simulink model "Arizona_base_NI"  (R2016b)
settings: Solver=FixedStepDiscrete  StartTime=0.0  StopTime=inf  FixedStep=Ts  RelTol=1e-3  EnableMultiTasking=on
undefined symbols (not defined in the file): DiscIntNeverNeededParam, N_ref, NInit, phiInit, xInit, yInit
libraries: xpcnilib x15, simulink x9, cstblocks x3
settings Model: SimulationMode=external  ExtModeTrigDuration=5  Creator=JBolder  LastModifiedBy=Arizona
settings SolverCC: EnableConcurrentExecution=on
settings DataIOCC: LimitDataPoints=on  SaveFormat=Array
settings OptimizationCC: BlockReduction=off  OptimizeBlockIOStorage=off  BufferReuse=off  GlobalBufferReuse=off  ExpressionFolding=off  LocalBlockOutputs=off  LifeSpan=inf
settings DebuggingCC: SolverPrmCheckMsg=warning  SFUnexpectedBacktrackingDiag=warning  SFNoUnconditionalDefaultTransitionDiag=warning  SFExecutionAtInitializationDiag=none
settings HardwareCC: ProdBitPerPointer=32  ProdBitPerSizeT=32  ProdBitPerPtrDiffT=32  ProdLargestAtomicFloat=None  ProdWordSize=32  ProdLongLongMode=on  ProdHWDeviceType=Generic->32-bit x86 compatible
settings ModelReferenceCC: PropagateSignalLabelsOutOfModel=off
settings RTWCC: SystemTargetFile=slrt.tlc  TemplateMakefile=slrt_default_tmf  Description=Simulink Real-Time  CodeExecutionProfiling=on  RTWCompilerOptimization=on
settings SimulinkRealTimeCC: xPCTargetPCEnvName=ArizonaTarget
settings ConfigComp: CovMetricSettings=dw  CovHtmlReporting=on  CovSaveCumulativeToWorkspaceVar=on  CovSaveSingleToWorkspaceVar=on  CovExternalEMLEnable=off  CovSFcnEnable=off

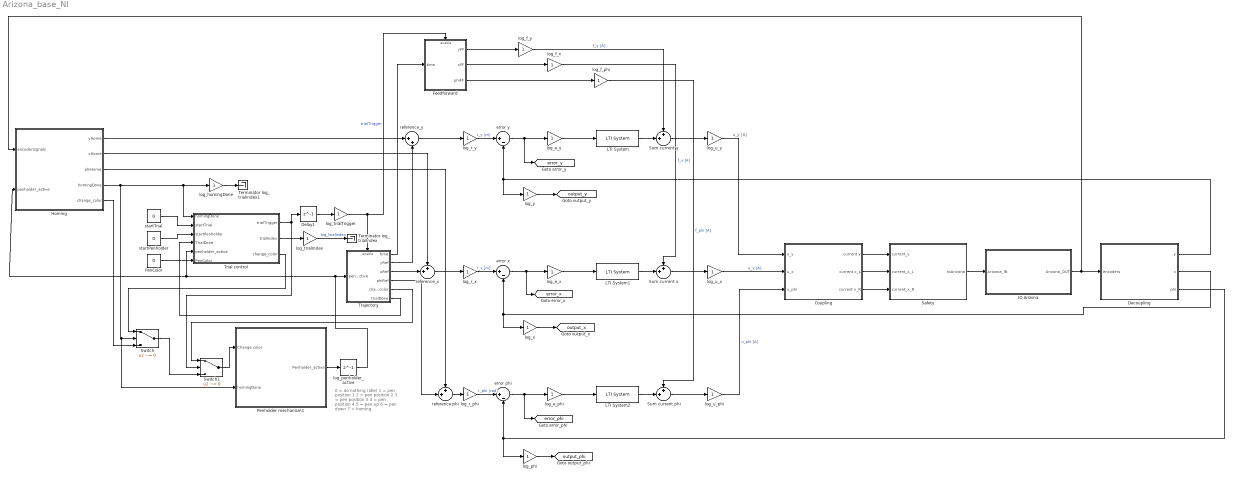
== system Arizona_base_NI ==
  note: u_y [A]
  note: 0 = do nothing (idle)
      | 1 = pen position 1
      | 2 = pen position 2
      | 3 = pen position 3
      | 4 = pen position 4
      | 5 = pen up
      | 6 = pen down
      | 7 = homing
  Coupling : Subsystem
  Decoupling : Subsystem
  Delay1 : Delay  DelayLength=1  InitialCondition=0
  Feedforward : Subsystem
  Homing : Subsystem
  IO Arizona : Subsystem
  LTI System : cstblocks/LTI System  sys=Cy  IC=[]
  LTI System1 : cstblocks/LTI System  sys=Cx  IC=[]
  LTI System2 : cstblocks/LTI System  sys=Cphi  IC=[]
  PenColor : Constant  Value=0
  Penholder mechanism1 : Subsystem
  Safety : Subsystem
  Sum current phi : Sum  Inputs=++|
  Sum current x : Sum  Inputs=++|
  Sum current y : Sum  Inputs=++|
  Switch : Switch  Criteria=u2 ~= 0
  Switch1 : Switch  Criteria=u2 ~= 0
  Terminator log_trialIndex : Terminator
  Terminator log_trialIndex1 : Terminator
  Trajectory : Subsystem  TreatAsAtomicUnit=on
  Trial control : Stateflow chart  TreatAsAtomicUnit=on
  error phi : Sum  Inputs=|+-
  error x : Sum  Inputs=|+-
  error y : Sum  Inputs=|+-
  log_e_phi : Gain
  log_e_x : Gain
  log_e_y : Gain
  log_f_phi : Gain
  log_f_x : Gain
  log_f_y : Gain
  log_homingDone : Gain
  log_penholder_active : Delay  DelayLength=1  InitialCondition=0
  log_phi : Gain
  log_r_phi : Gain
  log_r_x : Gain
  log_r_y : Gain
  log_trialIndex : Gain
  log_trialTrigger : Gain
  log_u_phi : Gain
  log_u_x : Gain
  log_u_y : Gain
  log_x : Gain
  log_y : Gain
  reference phi : Sum  Inputs=++|
  reference_x : Sum  Inputs=++|
  reference_y : Sum  Inputs=|++
  startPenholder : Constant  Value=0
  startTrial : Constant  Value=0
  tag scope: error_phi=global, error_x=global, error_y=global, output_phi=global, output_x=global, output_y=global
  wires:
  Decoupling/2(x) -> log_x/1, error x/2
  error x/1 -> log_e_x/1, [error_x]
  IO Arizona/1(Arizona_OUT) -> Decoupling/1(encoders), Homing/1(encoderSignals)
  error phi/1 -> log_e_phi/1, [error_phi]
  Homing/1(yHome) -> reference_y/1
  reference_y/1 -> log_r_y/1
  reference_x/1 -> log_r_x/1
  reference phi/1 -> log_r_phi/1
  Safety/1(toArizona) -> IO Arizona/1(Arizona_IN)
  Sum current phi/1 -> log_u_phi/1
  Trajectory/2(yRef) -> reference_y/2
  Trajectory/3(xRef) -> reference_x/2
  Trajectory/4(phiRef) -> reference phi/2
  error y/1 -> log_e_y/1, [error_y]
  Homing/3(phiHome) -> reference phi/1
  Homing/2(xHome) -> reference_x/1
  Homing/4(homingDone) -> Trial control/1(homingDone), log_homingDone/1, Penholder mechanism1/2(homingDone), Switch/2
  Trial control/1(trialTrigger) -> Switch1/2, Delay1/1
  startTrial/1 -> Trial control/2(startTrial)
  Trial control/2(trialIndex) -> log_trialIndex/1
  log_trialIndex/1 -> Terminator log_trialIndex/1  "log_trialIndex"
  log_trialTrigger/1 -> Feedforward/Enable, Trajectory/Enable  "trialTrigger"
  Feedforward/1(yFF) -> log_f_y/1
  log_e_y/1 -> LTI System/1
  Sum current y/1 -> log_u_y/1
  log_homingDone/1 -> Terminator log_trialIndex1/1
  log_r_y/1 -> error y/1  "r_y [m]"
  log_f_y/1 -> Sum current y/1  "f_y [A]"
  Feedforward/2(xFF) -> log_f_x/1
  log_f_x/1 -> Sum current x/1  "f_x [A]"
  log_r_x/1 -> error x/1  "r_x [m]"
  log_r_phi/1 -> error phi/1  "r_phi [rad]"
  log_f_phi/1 -> Sum current phi/1  "f_phi [A]"
  Feedforward/3(phiFF) -> log_f_phi/1
  log_u_y/1 -> Coupling/1(u_y)
  Sum current x/1 -> log_u_x/1
  Coupling/2(current x_L) -> Safety/2(current_x_L)
  Coupling/3(current x_R) -> Safety/3(current_x_R)
  Coupling/1(current y) -> Safety/1(current_y)
  Decoupling/1(y) -> log_y/1, error y/2
  Decoupling/3(phi) -> log_phi/1, error phi/2
  log_u_x/1 -> Coupling/2(u_x)  "u_x [A]"
  log_u_phi/1 -> Coupling/3(u_phi)  "u_phi [A]"
  log_penholder_active/1 -> Trajectory/1(penholder_active), Homing/2(penholder_active), Trial control/5(penholder_active)
  Trajectory/1(time) -> Feedforward/1(time)
  startPenholder/1 -> Trial control/3(startPenholder)
  Homing/5(change_color) -> Switch/3
  Switch1/1 -> Penholder mechanism1/1(Change color)
  Switch/1 -> Switch1/3
  Trajectory/6(trialDone) -> Trial control/4(TrialDone)
  Penholder mechanism1/1(Penholder_active) -> log_penholder_active/1
  Delay1/1 -> log_trialTrigger/1
  Trial control/3(change_color) -> Switch/1
  Trajectory/5(change_color) -> Switch1/1
  LTI System/1 -> Sum current y/2
  log_e_x/1 -> LTI System1/1
  LTI System1/1 -> Sum current x/2
  log_e_phi/1 -> LTI System2/1
  LTI System2/1 -> Sum current phi/2
  PenColor/1 -> Trial control/6(PenColor)
  log_y/1 -> [output_y]
  log_x/1 -> [output_x]
  log_phi/1 -> [output_phi]

== system Arizona_base_NI/Coupling ==
  u_y : Inport
  u_x : Inport  Port=2
  u_phi : Inport  Port=3
  Gain on u_phi : Gain  Gain=1/2.62
  Gain on u_x : Gain  Gain=1/2
  Sum current x_L : Sum  Inputs=|+-
  Sum current x_R : Sum  Inputs=++|
  current y : Outport
  current x_L : Outport  Port=2
  current x_R : Outport  Port=3
  wires:
  u_y/1 -> current y/1
  u_x/1 -> Gain on u_x/1
  Gain on u_phi/1 -> Sum current x_L/2, Sum current x_R/2
  Sum current x_L/1 -> current x_L/1
  Sum current x_R/1 -> current x_R/1
  u_phi/1 -> Gain on u_phi/1
  Gain on u_x/1 -> Sum current x_L/1, Sum current x_R/1

== system Arizona_base_NI/Decoupling ==
  encoders : Inport
  Bus Selector : BusSelector  OutputSignals=Encoders 6602/6229.encoder carriage,Encoders 6602/6229.encoder gantry x_L,Encoders 6602/6229.encoder gantry x_R
  Gain phi : Gain  Gain=1/2.62  OutDataTypeStr=double
  Gain x : Gain  Gain=1/2  OutDataTypeStr=double
  Sum x_L + x_R : Sum  Inputs=|++
  Sum x_R - x_L : Sum  Inputs=-+|
  y : Outport
  x : Outport  Port=2
  phi : Outport  Port=3
  wires:
  encoders/1 -> Bus Selector/1
  Bus Selector/3 -> Sum x_L + x_R/2, Sum x_R - x_L/2  "<encoder gantry x_R>"
  Bus Selector/2 -> Sum x_R - x_L/1, Sum x_L + x_R/1  "<encoder gantry x_L>"
  Sum x_L + x_R/1 -> Gain x/1
  Sum x_R - x_L/1 -> Gain phi/1
  Gain x/1 -> x/1
  Bus Selector/1 -> y/1  "<encoder carriage>"
  Gain phi/1 -> phi/1

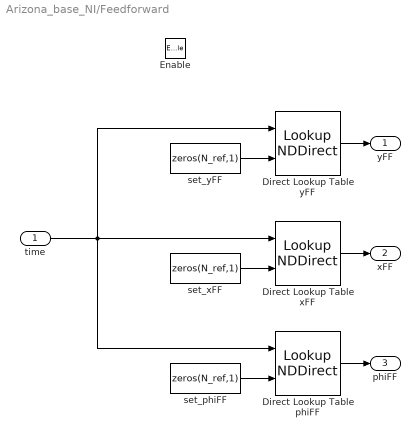
== system Arizona_base_NI/Feedforward ==
  time : Inport
  Enable : EnablePort  StatesWhenEnabling=reset
  Direct Lookup Table phiFF : LookupNDDirect  NumberOfTableDimensions=1  TableIsInput=on  Table=[4 5 ;16 19 ]
  Direct Lookup Table xFF : LookupNDDirect  NumberOfTableDimensions=1  TableIsInput=on  Table=[4 5 ;16 19 ]
  Direct Lookup Table yFF : LookupNDDirect  NumberOfTableDimensions=1  TableIsInput=on  Table=[4 5 ;16 19 ]
  set_phiFF : Constant  Value=zeros(N_ref,1)
  set_xFF : Constant  Value=zeros(N_ref,1)
  set_yFF : Constant  Value=zeros(N_ref,1)
  yFF : Outport
  xFF : Outport  Port=2
  phiFF : Outport  Port=3
  wires:
  Direct Lookup Table phiFF/1 -> phiFF/1
  Direct Lookup Table yFF/1 -> yFF/1
  Direct Lookup Table xFF/1 -> xFF/1
  set_yFF/1 -> Direct Lookup Table yFF/2
  set_xFF/1 -> Direct Lookup Table xFF/2
  time/1 -> Direct Lookup Table yFF/1, Direct Lookup Table xFF/1, Direct Lookup Table phiFF/1
  set_phiFF/1 -> Direct Lookup Table phiFF/2

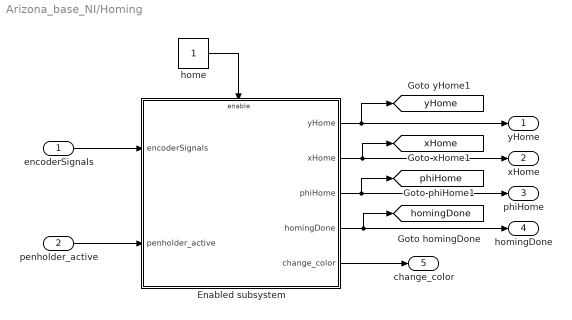
== system Arizona_base_NI/Homing ==
  encoderSignals : Inport
  penholder_active : Inport  Port=2
  Enabled subsystem : Subsystem
  home : Constant
  yHome : Outport
  xHome : Outport  Port=2
  phiHome : Outport  Port=3
  homingDone : Outport  Port=4
  change_color : Outport  Port=5
  tag scope: homingDone=global, phiHome=global, xHome=global, yHome=global
  wires:
  encoderSignals/1 -> Enabled subsystem/1(encoderSignals)
  Enabled subsystem/4(homingDone) -> homingDone/1, [homingDone]
  Enabled subsystem/2(xHome) -> xHome/1, [xHome]
  Enabled subsystem/1(yHome) -> [yHome], yHome/1
  Enabled subsystem/3(phiHome) -> [phiHome], phiHome/1
  home/1 -> Enabled subsystem/Enable
  penholder_active/1 -> Enabled subsystem/2(penholder_active)
  Enabled subsystem/5(change_color) -> change_color/1

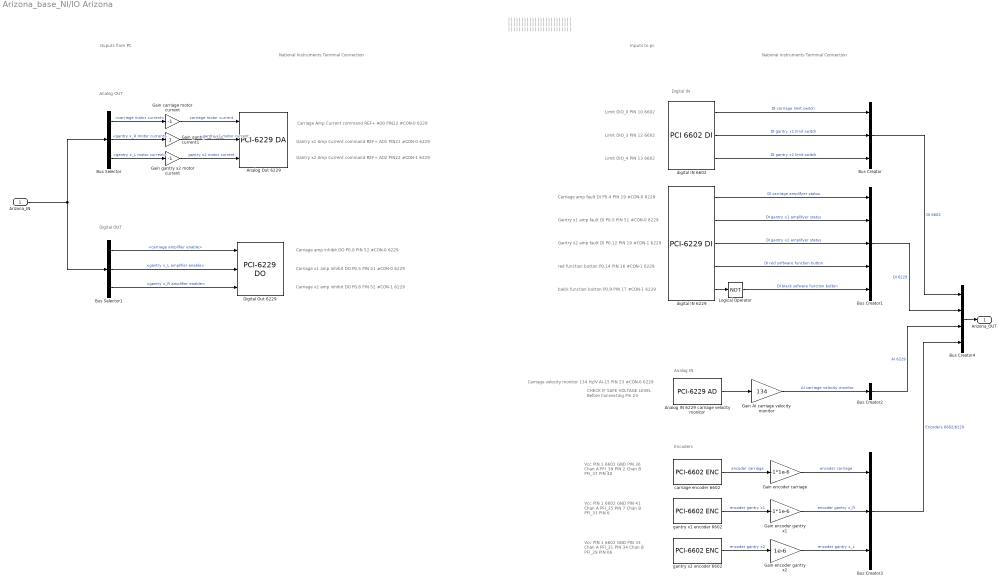
== system Arizona_base_NI/IO Arizona ==
  note: balck function button P0.9 PIN 17 #CON-1 6229
  note: Inputs to pc
  note: Digital OUT
  note: Analog OUT
  note: Analog IN
  note: Digital IN
  note: Gantry x2 amp fault DI P0.12 PIN 19 #CON-1 6229
  note: Carriage x2 amp inhibit DO P0.8 PIN 52 #CON-1 6229
  note: Gantry x2 Amp Current command REF+ AO2 PIN22 #CON-1 6229
  note: Gantry x1 amp fault DI P0.5 PIN 51 #CON-0 6229
  note: Carriage x1 amp inhibit DO P0.5 PIN 51 #CON-0 6229
  note: Gantry x1 Amp Current command REF+ AO1 PIN21 #CON-0 6229
  note: Vcc PIN 1		6602
      | GND PIN 33
      | Chan A PFI_31 PIN 34
      | Chan B PFI_29 PIN 66
  note: Limit DIO_4 PIN 13 6602
  note: Vcc PIN 1		6602
      | GND PIN 41
      | Chan A PFI_35 PIN 7
      | Chan B PFI_33 PIN 6
  note: Limit DIO_3 PIN 12 6602
  note: National Instruments Terminal Connection
  note: Carriage amp fault DI P0.4 PIN 19 #CON-0 6229
  note: Ouputs from PC
  note: CHECK IF SAFE VOLTAGE LEVEL
      | Before Connecting Pin 23
  note: Vcc PIN 1		6602
      | GND PIN 36
      | Chan A PFI_39 PIN 2
      | Chan B PFI_37 PIN 40
  note: Limit DIO_0 PIN 10 6602
  note: Carriage amp inhibit DO P0.0 PIN 52 #CON-0 6229
  note: Carriage velocity monitor 134 Hz/V AI-15 PIN 23 #CON-0 6229
  note: Carriage Amp Current command REF+ AO0 PIN22 #CON-0 6229
  note: National Instruments Terminal Connection
  note: |
      | |
      | |
      | |
      | |
      | |
      | |
      | |
      | |
      | |
      | |
      | |
      | |
      | |
      | |
      | |
      | |
      | |
      | |
      | |
      | |
      | |
      | |
      | |
      | |
      | |
      | |
      | |
      | |
      | |
      | |
      | |
      | |
      | |
      | |
      | |
      | |
      | |
      | |
      | |
      | |
      | |
      | |
      | |
      | |
      | |
      | |
      | |
      | |
      | |
      | |
      | |
      | |
      | |
      | |
      | |
      | |
      | |
      | |
      | |
      | |
      | |
      | |
      | |
      | |
      | |
      | |
      | |
      | |
      | |
      | |
      | |
  note: Encoders
  note: red function button P0.14 PIN 16 #CON-1 6229
  Arizona_IN : Inport
  Analog IN 6229 carriage velocity monitor : xpcnilib/A//D/M Series/PCI-6229 AD  channel=[16]  range=[10]  coupling=[0]  scantime=5e-6  sampletime=Ts  slot=-1
  Analog Out 6229 : xpcnilib/D//A/M Series/PCI-6229 DA  channel=[1 2 3]  reset=[1]  initValue=[0]  sampletime=Ts  slot=-1
  Bus Creator : BusCreator  Inputs=3
  Bus Creator1 : BusCreator  Inputs=5
  Bus Creator2 : BusCreator  Inputs=1
  Bus Creator3 : BusCreator  Inputs=3
  Bus Creator4 : BusCreator  Inputs=4
  Bus Selector : BusSelector  OutputSignals=carriage motor current,gantry x_R motor current,gantry x_L motor current
  Bus Selector1 : BusSelector  OutputSignals=carriage amplifier enable,gantry x_L amplifier enable,gantry x_R amplifier enable
  Digital Out 6229 : xpcnilib/Digital Output/M Series/PCI-6229 DO  channel=[1 6 9]  reset=[1]  initValue=[0]  sampletime=Ts  slot=-1
  Gain AI carriage velocity monitor : Gain  Gain=134
  Gain carriage motor current : Gain  Gain=-1
  Gain encoder carriage : Gain  Gain=-1*1e-6
  Gain encoder gantry x1 : Gain  Gain=-1*1e-6
  Gain encoder gantry x2 : Gain  Gain=1e-6
  Gain gantry x2 motor current : Gain  Gain=-1
  Gain gantry x2 motor current1 : Gain
  Logical Operator : Logic  Operator=NOT  AllPortsSameDT=off  OutDataTypeStr=boolean
  carriage encoder 6602 : xpcnilib/Incremental Encoder/PCI-6602 ENC  channel=1  countMode=Quadrature Mode X4  initCount=0  reload=off  indexPhase=A low B low  filter=None  sampleTime=Ts  slot=-1
  digital IN 6229 : xpcnilib/Digital Input/M Series/PCI-6229 DI  channel=[5 2 13 15 10]  sampletime=Ts  slot=-1
  digital IN 6602 : xpcnilib/Digital Input/PCI 6602 DI   channel=[1 4 5]  tsamp=Ts  slot=-1
  gantry x1 encoder 6602 : xpcnilib/Incremental Encoder/PCI-6602 ENC  channel=2  countMode=Quadrature Mode X4  initCount=0  reload=off  indexPhase=A low B low  filter=None  sampleTime=Ts  slot=-1
  gantry x2 encoder 6602 : xpcnilib/Incremental Encoder/PCI-6602 ENC  channel=3  countMode=Quadrature Mode X4  initCount=0  reload=off  indexPhase=A low B low  filter=None  sampleTime=Ts  slot=-1
  Arizona_OUT : Outport
  wires:
  digital IN 6602/3 -> Bus Creator/3  "DI gantry x2 limit switch"
  Arizona_IN/1 -> Bus Selector/1, Bus Selector1/1
  Bus Creator3/1 -> Bus Creator4/4  "Encoders 6602/6229"
  Bus Creator2/1 -> Bus Creator4/3  "AI 6229"
  Bus Creator1/1 -> Bus Creator4/2  "DI 6229"
  Bus Creator/1 -> Bus Creator4/1  "DI 6602"
  Gain carriage motor current/1 -> Analog Out 6229/1  "carriage motor current"
  Bus Selector/3 -> Gain gantry x2 motor current/1  "<gantry x_L motor current>"
  Bus Selector1/3 -> Digital Out 6229/3  "<gantry x_R amplifier enable>"
  digital IN 6229/5 -> Logical Operator/1
  Logical Operator/1 -> Bus Creator1/5  "DI black sofware function button"
  digital IN 6229/2 -> Bus Creator1/2  "DI gantry x1 amplifyer status"
  digital IN 6229/3 -> Bus Creator1/3  "DI gantry x2 amplifyer status"
  Bus Selector/2 -> Gain gantry x2 motor current1/1  "<gantry x_R motor current>"
  Gain encoder carriage/1 -> Bus Creator3/1  "encoder carriage"
  Bus Selector1/2 -> Digital Out 6229/2  "<gantry x_L amplifier enable>"
  Bus Selector1/1 -> Digital Out 6229/1  "<carriage amplifier enable>"
  gantry x1 encoder 6602/1 -> Gain encoder gantry x1/1  "encoder gantry x1"
  digital IN 6229/4 -> Bus Creator1/4  "DI red software function button"
  digital IN 6602/2 -> Bus Creator/2  "DI gantry x1 limit switch"
  Gain encoder gantry x1/1 -> Bus Creator3/2  "encoder gantry x_R"
  digital IN 6229/1 -> Bus Creator1/1  "DI carriage amplifyer status"
  digital IN 6602/1 -> Bus Creator/1  "DI carriage limit switch"
  Analog IN 6229 carriage velocity monitor/1 -> Gain AI carriage velocity monitor/1
  carriage encoder 6602/1 -> Gain encoder carriage/1  "encoder carriage"
  Bus Selector/1 -> Gain carriage motor current/1  "<carriage motor current>"
  gantry x2 encoder 6602/1 -> Gain encoder gantry x2/1  "encoder gantry x2"
  Gain gantry x2 motor current/1 -> Analog Out 6229/3  "gantry x2 motor current"
  Gain encoder gantry x2/1 -> Bus Creator3/3  "encoder gantry x_L"
  Gain AI carriage velocity monitor/1 -> Bus Creator2/1  "AI carriage velocity monitor"
  Bus Creator4/1 -> Arizona_OUT/1
  Gain gantry x2 motor current1/1 -> Analog Out 6229/2  "gantry x1 motor current"

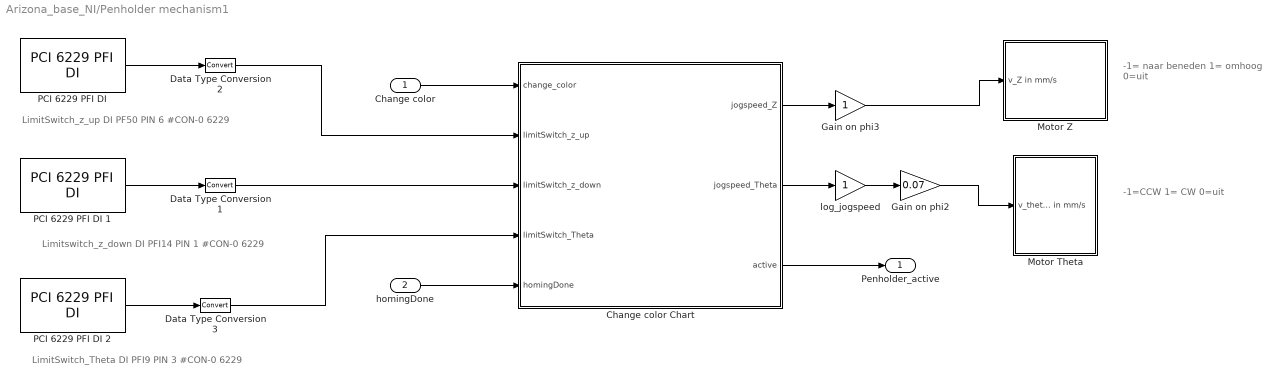
== system Arizona_base_NI/Penholder mechanism1 ==
  note: -1= naar beneden
      | 1= omhoog
      | 0=uit
  note: -1=CCW
      | 1= CW
      | 0=uit
  note: LimitSwitch_z_up DI PF50 PIN 6 #CON-0 6229
  note: Limitswitch_z_down DI PFI14 PIN 1 #CON-0 6229
  note: LimitSwitch_Theta DI PFI9 PIN 3 #CON-0 6229
  Change color : Inport
  homingDone : Inport  Port=2
  Change color Chart : Stateflow chart  TreatAsAtomicUnit=on
  Data Type Conversion1 : DataTypeConversion
  Data Type Conversion2 : DataTypeConversion
  Data Type Conversion3 : DataTypeConversion
  Gain on phi2 : Gain  Gain=0.07
  Gain on phi3 : Gain
  Motor Theta : Subsystem
  Motor Z : Subsystem
  "PCI 6229 PFI DI " : xpcnilib/Digital Input/M Series/PCI 6229 PFI DI   channel=[5]  sampleTime=Ts  slot=-1
  PCI 6229 PFI DI 1 : xpcnilib/Digital Input/M Series/PCI 6229 PFI DI   channel=[14]  sampleTime=Ts  slot=-1
  PCI 6229 PFI DI 2 : xpcnilib/Digital Input/M Series/PCI 6229 PFI DI   channel=[9]  sampleTime=Ts  slot=-1
  log_jogspeed : Gain
  Penholder_active : Outport
  wires:
  PCI 6229 PFI DI 1/1 -> Data Type Conversion1/1
  "PCI 6229 PFI DI "/1 -> Data Type Conversion2/1
  Gain on phi2/1 -> Motor Theta/1(v_theta in mm/s)
  Gain on phi3/1 -> Motor Z/1(v_Z in mm/s)
  PCI 6229 PFI DI 2/1 -> Data Type Conversion3/1
  Data Type Conversion3/1 -> Change color Chart/4(limitSwitch_Theta)
  Change color/1 -> Change color Chart/1(change_color)
  Change color Chart/1(jogspeed_Z) -> Gain on phi3/1
  Change color Chart/2(jogspeed_Theta) -> log_jogspeed/1
  Data Type Conversion2/1 -> Change color Chart/2(limitSwitch_z_up)
  Data Type Conversion1/1 -> Change color Chart/3(limitSwitch_z_down)
  Change color Chart/3(active) -> Penholder_active/1
  log_jogspeed/1 -> Gain on phi2/1
  homingDone/1 -> Change color Chart/5(homingDone)

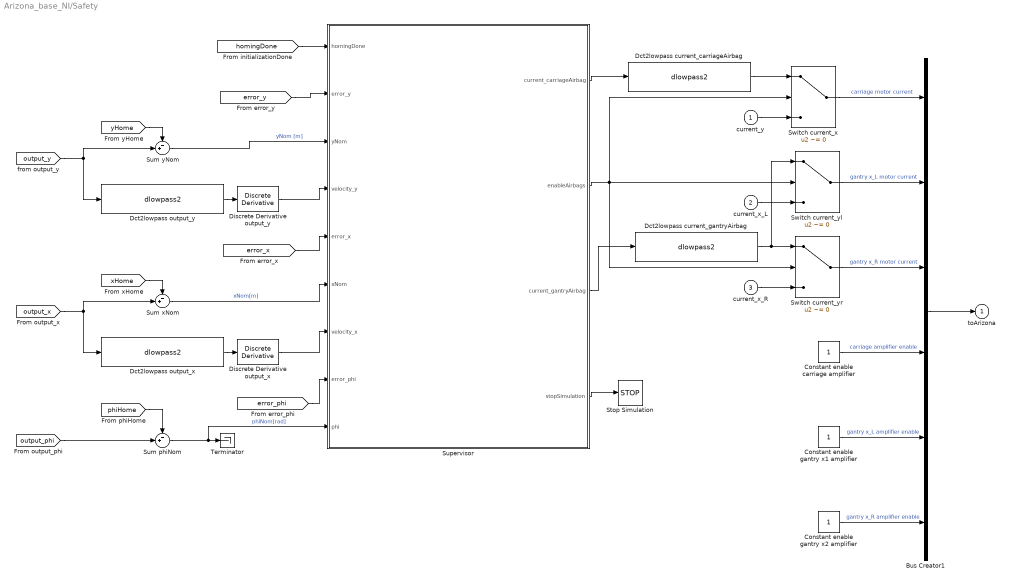
== system Arizona_base_NI/Safety ==
  current_y : Inport
  current_x_L : Inport  Port=2
  current_x_R : Inport  Port=3
  Bus Creator1 : BusCreator  Inputs='carriage motor current','gantry x_L motor current','gantry x_R motor current','carriage amplifier enable','gantry x_L amplifier enable','gantry x_R amplifier enable'
  Constant enable carriage amplifier : Constant
  Constant enable gantry x1 amplifier : Constant
  Constant enable gantry x2 amplifier : Constant
  Dct2lowpass current_carriageAirbag : S-Function  FunctionName=dlowpass2  Parameters=f_den, b_den, 0.001  SFunctionDeploymentMode=off  EnableBusSupport=off  mask(dctools){f_den=5, b_den=2}
      mask prompts: f_den "Pole [Hz]"; b_den "Damping pole [-]"
      mask help: This block implements a discrete time 2nd order lowpass filter.
      mask Display: disp('DCT 2nd order lowpass')
  Dct2lowpass current_gantryAirbag : S-Function  FunctionName=dlowpass2  Parameters=f_den, b_den, 0.001  SFunctionDeploymentMode=off  EnableBusSupport=off  mask(dctools){f_den=5, b_den=2}
      mask prompts: f_den "Pole [Hz]"; b_den "Damping pole [-]"
      mask help: This block implements a discrete time 2nd order lowpass filter.
      mask Display: disp('DCT 2nd order lowpass')
  Dct2lowpass output_x : S-Function  FunctionName=dlowpass2  Parameters=f_den, b_den, 0.001  SFunctionDeploymentMode=off  EnableBusSupport=off  mask(dctools){f_den=10, b_den=2}
      mask prompts: f_den "Pole [Hz]"; b_den "Damping pole [-]"
      mask help: This block implements a discrete time 2nd order lowpass filter.
      mask Display: disp('DCT 2nd order lowpass')
  Dct2lowpass output_y : S-Function  FunctionName=dlowpass2  Parameters=f_den, b_den, 0.001  SFunctionDeploymentMode=off  EnableBusSupport=off  mask(dctools){f_den=10, b_den=2}
      mask prompts: f_den "Pole [Hz]"; b_den "Damping pole [-]"
      mask help: This block implements a discrete time 2nd order lowpass filter.
      mask Display: disp('DCT 2nd order lowpass')
  Discrete Derivative output_x : simulink/Discrete/Discrete Derivative  gainval=1.0  ICPrevScaledInput=0.0  OutMin=[]  OutMax=[]  OutDataType=fixdt(1, 16)  OutScaling=2^-10  DoSatur=off
  Discrete Derivative output_y : simulink/Discrete/Discrete Derivative  gainval=1.0  ICPrevScaledInput=0.0  OutMin=[]  OutMax=[]  OutDataType=fixdt(1, 16)  OutScaling=2^-10  DoSatur=off
  Stop Simulation : Stop
  Sum phiNom : Sum  Inputs=-+|
  Sum xNom : Sum  Inputs=-+|
  Sum yNom : Sum  Inputs=-+|
  Supervisor : Stateflow chart  TreatAsAtomicUnit=on
  Switch current_x : Switch  Criteria=u2 ~= 0
  Switch current_yl : Switch  Criteria=u2 ~= 0
  Switch current_yr : Switch  Criteria=u2 ~= 0
  Terminator : Terminator
  toArizona : Outport
  wires:
  [phiHome] -> Sum phiNom/1
  Sum phiNom/1 -> Supervisor/9(phi), Terminator/1  "phiNom[rad]"
  current_x_L/1 -> Switch current_yl/3
  current_x_R/1 -> Switch current_yr/3
  Dct2lowpass current_carriageAirbag/1 -> Switch current_x/1
  Dct2lowpass current_gantryAirbag/1 -> Switch current_yl/1, Switch current_yr/1
  Supervisor/3(current_gantryAirbag) -> Dct2lowpass current_gantryAirbag/1
  Discrete Derivative output_x/1 -> Supervisor/7(velocity_x)
  [xHome] -> Sum xNom/1
  Dct2lowpass output_x/1 -> Discrete Derivative output_x/1
  Sum xNom/1 -> Supervisor/6(xNom)  "xNom[m]"
  [output_x] -> Sum xNom/2, Dct2lowpass output_x/1
  [error_phi] -> Supervisor/8(error_phi)
  [error_x] -> Supervisor/5(error_x)
  Supervisor/2(enableAirbags) -> Switch current_yr/2, Switch current_yl/2, Switch current_x/2
  Supervisor/1(current_carriageAirbag) -> Dct2lowpass current_carriageAirbag/1
  Supervisor/4(stopSimulation) -> Stop Simulation/1
  [error_y] -> Supervisor/2(error_y)
  Switch current_x/1 -> Bus Creator1/1  "carriage motor current"
  [homingDone] -> Supervisor/1(homingDone)
  [yHome] -> Sum yNom/1
  current_y/1 -> Switch current_x/3
  Discrete Derivative output_y/1 -> Supervisor/4(velocity_y)
  Dct2lowpass output_y/1 -> Discrete Derivative output_y/1
  Sum yNom/1 -> Supervisor/3(yNom)  "yNom [m]"
  [output_y] -> Sum yNom/2, Dct2lowpass output_y/1
  Bus Creator1/1 -> toArizona/1
  Constant enable gantry x1 amplifier/1 -> Bus Creator1/5  "gantry x_L amplifier enable"
  Constant enable gantry x2 amplifier/1 -> Bus Creator1/6  "gantry x_R amplifier enable"
  Switch current_yl/1 -> Bus Creator1/2  "gantry x_L motor current"
  Constant enable carriage amplifier/1 -> Bus Creator1/4  "carriage amplifier enable"
  Switch current_yr/1 -> Bus Creator1/3  "gantry x_R motor current"
  [output_phi] -> Sum phiNom/2

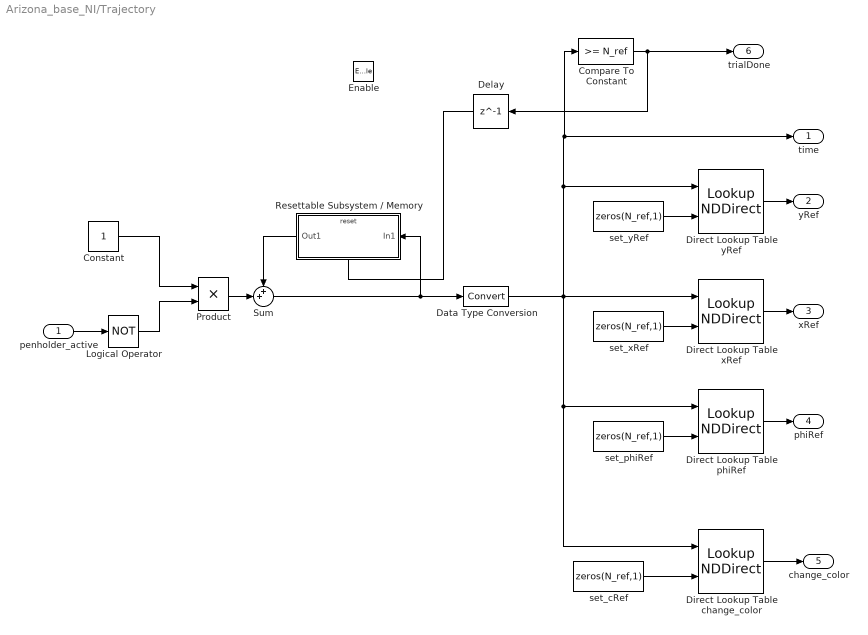
== system Arizona_base_NI/Trajectory ==
  penholder_active : Inport
  Enable : EnablePort  StatesWhenEnabling=reset
  Compare To Constant : simulink/Logic and Bit Operations/Compare To Constant  relop=>=  const=N_ref  OutDataTypeStr=boolean
  Constant : Constant
  Data Type Conversion : DataTypeConversion
  Delay : Delay  DelayLength=1  InitialCondition=0
  Direct Lookup Table change_color : LookupNDDirect  NumberOfTableDimensions=1  TableIsInput=on  Table=[4 5 ;16 19 ]
  Direct Lookup Table phiRef : LookupNDDirect  NumberOfTableDimensions=1  TableIsInput=on  Table=[4 5 ;16 19 ]
  Direct Lookup Table xRef : LookupNDDirect  NumberOfTableDimensions=1  TableIsInput=on  Table=[4 5 ;16 19 ]
  Direct Lookup Table yRef : LookupNDDirect  NumberOfTableDimensions=1  TableIsInput=on  Table=[4 5 ;16 19 ]
  Logical Operator : Logic  Operator=NOT  AllPortsSameDT=off  OutDataTypeStr=boolean
  Product : Product
  Resettable Subsystem / Memory : Subsystem  TreatAsAtomicUnit=on
  Sum : Sum  Inputs=++|
  set_cRef : Constant  Value=zeros(N_ref,1)
  set_phiRef : Constant  Value=zeros(N_ref,1)
  set_xRef : Constant  Value=zeros(N_ref,1)
  set_yRef : Constant  Value=zeros(N_ref,1)
  time : Outport
  yRef : Outport  Port=2
  xRef : Outport  Port=3
  phiRef : Outport  Port=4
  change_color : Outport  Port=5
  trialDone : Outport  Port=6
  wires:
  Direct Lookup Table phiRef/1 -> phiRef/1
  Direct Lookup Table yRef/1 -> yRef/1
  Direct Lookup Table xRef/1 -> xRef/1
  set_yRef/1 -> Direct Lookup Table yRef/2
  set_xRef/1 -> Direct Lookup Table xRef/2
  Data Type Conversion/1 -> Compare To Constant/1, time/1, Direct Lookup Table yRef/1, Direct Lookup Table xRef/1, Direct Lookup Table change_color/1, Direct Lookup Table phiRef/1
  set_phiRef/1 -> Direct Lookup Table phiRef/2
  Constant/1 -> Product/1
  Sum/1 -> Resettable Subsystem / Memory/1(In1), Data Type Conversion/1
  penholder_active/1 -> Logical Operator/1
  Logical Operator/1 -> Product/2
  Direct Lookup Table change_color/1 -> change_color/1
  set_cRef/1 -> Direct Lookup Table change_color/2
  Compare To Constant/1 -> Delay/1, trialDone/1
  Product/1 -> Sum/2
  Resettable Subsystem / Memory/1(Out1) -> Sum/1
  Delay/1 -> Resettable Subsystem / Memory/Reset

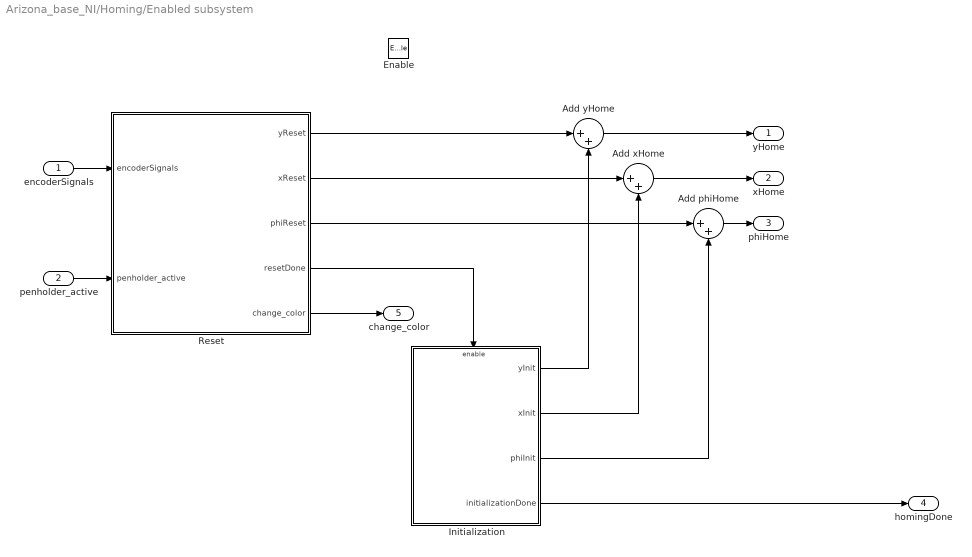
== system Arizona_base_NI/Homing/Enabled subsystem ==
  encoderSignals : Inport
  penholder_active : Inport  Port=2
  Enable : EnablePort  StatesWhenEnabling=reset
  Add phiHome : Sum  Inputs=|++
  Add xHome : Sum  Inputs=|++
  Add yHome : Sum  Inputs=|++
  Initialization : Subsystem  TreatAsAtomicUnit=on
  Reset : Subsystem
  yHome : Outport
  xHome : Outport  Port=2
  phiHome : Outport  Port=3
  homingDone : Outport  Port=4  InitialOutput=1
  change_color : Outport  Port=5
  wires:
  encoderSignals/1 -> Reset/1(encoderSignals)
  Reset/4(resetDone) -> Initialization/Enable
  Reset/1(yReset) -> Add yHome/1
  Reset/2(xReset) -> Add xHome/1
  Reset/3(phiReset) -> Add phiHome/1
  Initialization/4(initializationDone) -> homingDone/1
  Add xHome/1 -> xHome/1
  Add yHome/1 -> yHome/1
  Add phiHome/1 -> phiHome/1
  penholder_active/1 -> Reset/2(penholder_active)
  Reset/5(change_color) -> change_color/1
  Initialization/3(phiInit) -> Add phiHome/2
  Initialization/1(yInit) -> Add yHome/2
  Initialization/2(xInit) -> Add xHome/2

== system Arizona_base_NI/Penholder mechanism1/Motor Theta ==
  note: enable DO PFI4 PIN 41 #CON-0 6229
  note: direction DO PFI3 PIN 42 #CON-0 6229
  v_theta in mm/s : Inport
  Abs : Abs
  Compare To Zero : simulink/Logic and Bit Operations/Compare To Zero  relop=>  OutDataTypeStr=boolean
  Data Type Conversion : DataTypeConversion
  "PCI 6229 PFI DO " : xpcnilib/Digital Output/M Series/PCI 6229 PFI DO   channel=[3,4]  reset=[1]  initial=[0]  sampleTime=-1  slot=-1
  PCI 6229 PWM Generate Chan 0 : xpcnilib/Counter/M Series/PCI 6229 PWM Generate   channel=0  initHigh=0  initLow=4000  arm=off  disarmlevel=Disarm to LOW  stoplevel=Stop to LOW  sampletime=-1  slot=-1
  PWMcreator5 : Subsystem
  wires:
  PWMcreator5/1(HighSamples) -> PCI 6229 PWM Generate Chan 0/1
  PWMcreator5/2(LowSamples) -> PCI 6229 PWM Generate Chan 0/2
  Compare To Zero/1 -> Data Type Conversion/1
  PWMcreator5/3(DirectionBit) -> "PCI 6229 PFI DO "/1
  Data Type Conversion/1 -> "PCI 6229 PFI DO "/2
  Abs/1 -> Compare To Zero/1
  v_theta in mm/s/1 -> Abs/1, PWMcreator5/1(velocity [mm / s])

== system Arizona_base_NI/Penholder mechanism1/Motor Z ==
  note: enable DO PFI11 PIN 46 #CON-0 6229
  note: direction DO PFI10 PIN 45 #CON-0 6229
  v_Z in mm/s : Inport
  Abs1 : Abs
  Compare To Zero1 : simulink/Logic and Bit Operations/Compare To Zero  relop=>  OutDataTypeStr=boolean
  Data Type Conversion1 : DataTypeConversion
  PCI 6229 PFI DO 1 : xpcnilib/Digital Output/M Series/PCI 6229 PFI DO   channel=[10,11]  reset=[1]  initial=[0]  sampleTime=-1  slot=-1
  PCI 6229 PWM Generate Chan 1 : xpcnilib/Counter/M Series/PCI 6229 PWM Generate   channel=1  initHigh=0  initLow=4000  arm=off  disarmlevel=Disarm to LOW  stoplevel=Stop to LOW  sampletime=-1  slot=-1
  PWMcreator1 : Subsystem
  wires:
  PWMcreator1/1(HighSamples) -> PCI 6229 PWM Generate Chan 1/1
  PWMcreator1/2(LowSamples) -> PCI 6229 PWM Generate Chan 1/2
  Compare To Zero1/1 -> Data Type Conversion1/1
  PWMcreator1/3(DirectionBit) -> PCI 6229 PFI DO 1/1
  v_Z in mm/s/1 -> Abs1/1, PWMcreator1/1(velocity [mm / s])
  Data Type Conversion1/1 -> PCI 6229 PFI DO 1/2
  Abs1/1 -> Compare To Zero1/1

== system Arizona_base_NI/Trajectory/Resettable Subsystem // Memory ==
  In1 : Inport
  Reset : ResetPort  DisableCoverage=on
  Memory : Memory
  Out1 : Outport
  wires:
  In1/1 -> Memory/1
  Memory/1 -> Out1/1

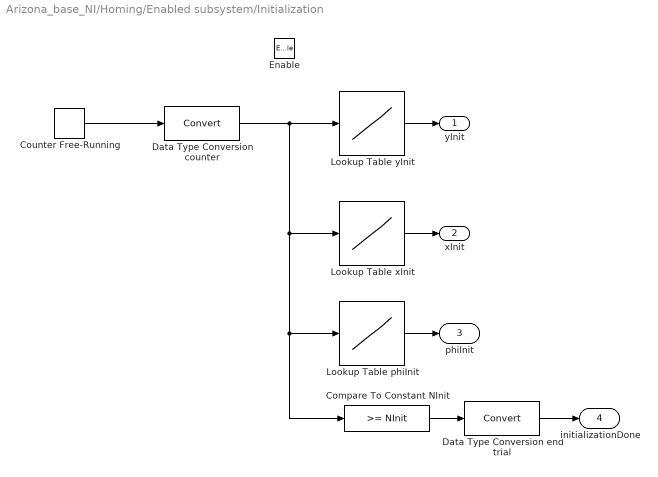
== system Arizona_base_NI/Homing/Enabled subsystem/Initialization ==
  Enable : EnablePort
  Compare To Constant NInit : simulink/Logic and Bit Operations/Compare To Constant  relop=>=  const=NInit  OutDataTypeStr=boolean
  Counter Free-Running : simulink/Sources/Counter Free-Running  NumBits=32  tsamp=-1
  Data Type Conversion counter : DataTypeConversion
  Data Type Conversion end trial : DataTypeConversion
  Lookup Table phiInit : Lookup_n-D  NumberOfTableDimensions=1  BreakpointsForDimension1=0:length(phiInit)-1  IndexSearchMethod=Evenly spaced points  Table=phiInit  InterpMethod=Flat  ExtrapMethod=Clip  InternalRulePriority=Speed  RndMeth=Simplest  InputSameDT=on
  Lookup Table xInit : Lookup_n-D  NumberOfTableDimensions=1  BreakpointsForDimension1=0:length(xInit)-1  IndexSearchMethod=Evenly spaced points  Table=xInit  InterpMethod=Flat  ExtrapMethod=Clip  InternalRulePriority=Speed  RndMeth=Simplest  InputSameDT=on
  Lookup Table yInit : Lookup_n-D  NumberOfTableDimensions=1  BreakpointsForDimension1=0:length(yInit)-1  IndexSearchMethod=Evenly spaced points  Table=yInit  InterpMethod=Flat  ExtrapMethod=Clip  InternalRulePriority=Speed  RndMeth=Simplest  InputSameDT=on
  yInit : Outport
  xInit : Outport  Port=2
  phiInit : Outport  Port=3
  initializationDone : Outport  Port=4
  wires:
  Data Type Conversion end trial/1 -> initializationDone/1
  Compare To Constant NInit/1 -> Data Type Conversion end trial/1
  Lookup Table phiInit/1 -> phiInit/1
  Lookup Table xInit/1 -> xInit/1
  Data Type Conversion counter/1 -> Lookup Table yInit/1, Compare To Constant NInit/1, Lookup Table phiInit/1, Lookup Table xInit/1
  Counter Free-Running/1 -> Data Type Conversion counter/1
  Lookup Table yInit/1 -> yInit/1

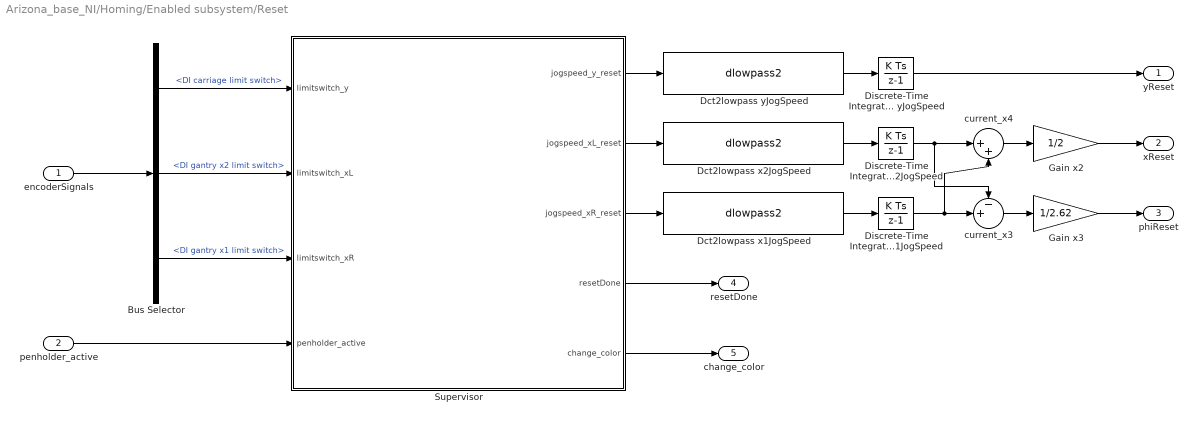
== system Arizona_base_NI/Homing/Enabled subsystem/Reset ==
  encoderSignals : Inport
  penholder_active : Inport  Port=2
  Bus Selector : BusSelector  OutputSignals=DI 6602.DI carriage limit switch,DI 6602.DI gantry x2 limit switch,DI 6602.DI gantry x1 limit switch
  Dct2lowpass x1JogSpeed : S-Function  FunctionName=dlowpass2  Parameters=f_den, b_den, 0.001  SFunctionDeploymentMode=off  EnableBusSupport=off  mask(dctools){f_den=20, b_den=2}
      mask prompts: f_den "Pole [Hz]"; b_den "Damping pole [-]"
      mask help: This block implements a discrete time 2nd order lowpass filter.
      mask Display: disp('DCT 2nd order lowpass')
  Dct2lowpass x2JogSpeed : S-Function  FunctionName=dlowpass2  Parameters=f_den, b_den, 0.001  SFunctionDeploymentMode=off  EnableBusSupport=off  mask(dctools){f_den=20, b_den=2}
      mask prompts: f_den "Pole [Hz]"; b_den "Damping pole [-]"
      mask help: This block implements a discrete time 2nd order lowpass filter.
      mask Display: disp('DCT 2nd order lowpass')
  Dct2lowpass yJogSpeed : S-Function  FunctionName=dlowpass2  Parameters=f_den, b_den, 0.001  SFunctionDeploymentMode=off  EnableBusSupport=off  mask(dctools){f_den=10, b_den=1}
      mask prompts: f_den "Pole [Hz]"; b_den "Damping pole [-]"
      mask help: This block implements a discrete time 2nd order lowpass filter.
      mask Display: disp('DCT 2nd order lowpass')
  Discrete-Time Integrator x1JogSpeed : DiscreteIntegrator  SampleTime=-1  ICPrevOutput=DiscIntNeverNeededParam  ICPrevScaledInput=DiscIntNeverNeededParam
  Discrete-Time Integrator x2JogSpeed : DiscreteIntegrator  SampleTime=-1  ICPrevOutput=DiscIntNeverNeededParam  ICPrevScaledInput=DiscIntNeverNeededParam
  Discrete-Time Integrator yJogSpeed : DiscreteIntegrator  SampleTime=-1  ICPrevOutput=DiscIntNeverNeededParam  ICPrevScaledInput=DiscIntNeverNeededParam
  Gain x2 : Gain  Gain=1/2  OutDataTypeStr=double
  Gain x3 : Gain  Gain=1/2.62  OutDataTypeStr=double
  Supervisor : Stateflow chart  TreatAsAtomicUnit=on
  current_x3 : Sum  Inputs=-+|
  current_x4 : Sum  Inputs=|++
  yReset : Outport
  xReset : Outport  Port=2
  phiReset : Outport  Port=3
  resetDone : Outport  Port=4
  change_color : Outport  Port=5
  wires:
  Bus Selector/3 -> Supervisor/3(limitswitch_xR)  "<DI gantry x1 limit switch>"
  Discrete-Time Integrator yJogSpeed/1 -> yReset/1
  Gain x2/1 -> xReset/1
  encoderSignals/1 -> Bus Selector/1
  Supervisor/4(resetDone) -> resetDone/1
  Supervisor/2(jogspeed_xL_reset) -> Dct2lowpass x2JogSpeed/1
  Supervisor/3(jogspeed_xR_reset) -> Dct2lowpass x1JogSpeed/1
  Dct2lowpass x2JogSpeed/1 -> Discrete-Time Integrator x2JogSpeed/1
  Dct2lowpass x1JogSpeed/1 -> Discrete-Time Integrator x1JogSpeed/1
  Bus Selector/2 -> Supervisor/2(limitswitch_xL)  "<DI gantry x2 limit switch>"
  Supervisor/1(jogspeed_y_reset) -> Dct2lowpass yJogSpeed/1
  Dct2lowpass yJogSpeed/1 -> Discrete-Time Integrator yJogSpeed/1
  Bus Selector/1 -> Supervisor/1(limitswitch_y)  "<DI carriage limit switch>"
  Discrete-Time Integrator x1JogSpeed/1 -> current_x4/2, current_x3/2
  Discrete-Time Integrator x2JogSpeed/1 -> current_x3/1, current_x4/1
  current_x4/1 -> Gain x2/1
  current_x3/1 -> Gain x3/1
  Gain x3/1 -> phiReset/1
  penholder_active/1 -> Supervisor/4(penholder_active)
  Supervisor/5(change_color) -> change_color/1

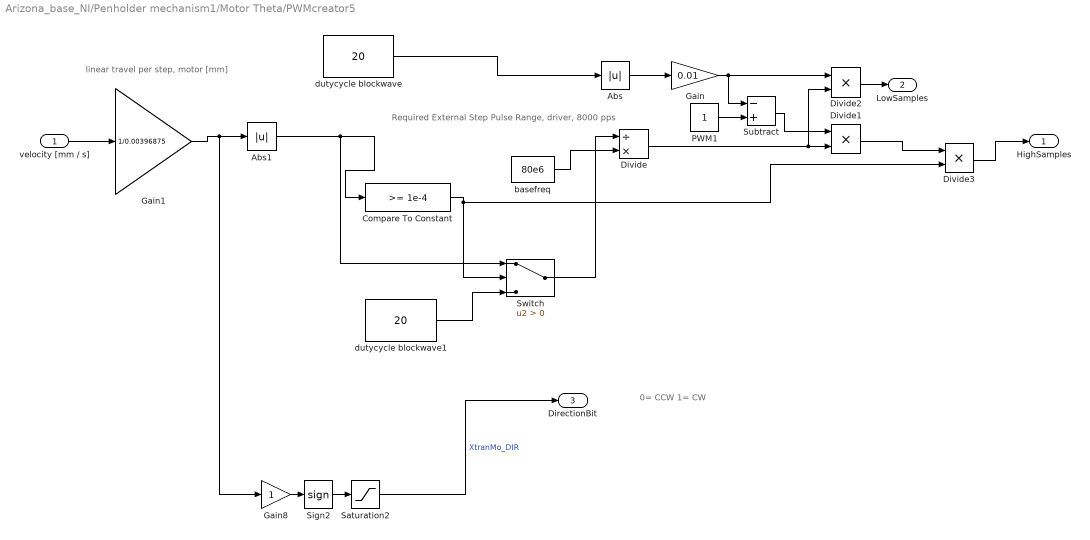
== system Arizona_base_NI/Penholder mechanism1/Motor Theta/PWMcreator5 ==
  note: Required External Step Pulse Range, driver, 8000 pps
  note: linear travel per step, motor [mm]
  note: 0= CCW
      | 1= CW
  velocity [mm / s] : Inport
  Abs : Abs
  Abs1 : Abs
  Compare To Constant : simulink/Logic and Bit Operations/Compare To Constant  relop=>=  const=1e-4  OutDataTypeStr=boolean
  Divide : Product  Inputs=/*
  Divide1 : Product  Inputs=**
  Divide2 : Product  Inputs=**
  Divide3 : Product  Inputs=**
  Gain : Gain  Gain=0.01
  Gain1 : Gain  Gain=1/0.00396875
  Gain8 : Gain
  PWM1 : Constant
  Saturation2 : Saturate  UpperLimit=1  LowerLimit=0
  Sign2 : Signum
  Subtract : Sum  Inputs=-+
  Switch : Switch  Criteria=u2 > Threshold
  basefreq : Constant  Value=80e6
  dutycycle blockwave : Constant  Value=20
  dutycycle blockwave1 : Constant  Value=20
  HighSamples : Outport
  LowSamples : Outport  Port=2
  DirectionBit : Outport  Port=3
  wires:
  Abs/1 -> Gain/1
  Sign2/1 -> Saturation2/1
  Gain8/1 -> Sign2/1
  Divide1/1 -> Divide3/1
  velocity [mm / s]/1 -> Gain1/1
  Divide2/1 -> LowSamples/1
  dutycycle blockwave/1 -> Abs/1
  PWM1/1 -> Subtract/2
  Subtract/1 -> Divide1/1
  Divide/1 -> Divide1/2, Divide2/2
  Gain/1 -> Subtract/1, Divide2/1
  basefreq/1 -> Divide/2
  Abs1/1 -> Compare To Constant/1, Switch/1
  Gain1/1 -> Gain8/1, Abs1/1
  Compare To Constant/1 -> Divide3/2, Switch/2
  Switch/1 -> Divide/1
  dutycycle blockwave1/1 -> Switch/3
  Divide3/1 -> HighSamples/1
  Saturation2/1 -> DirectionBit/1  "XtranMo_DIR"

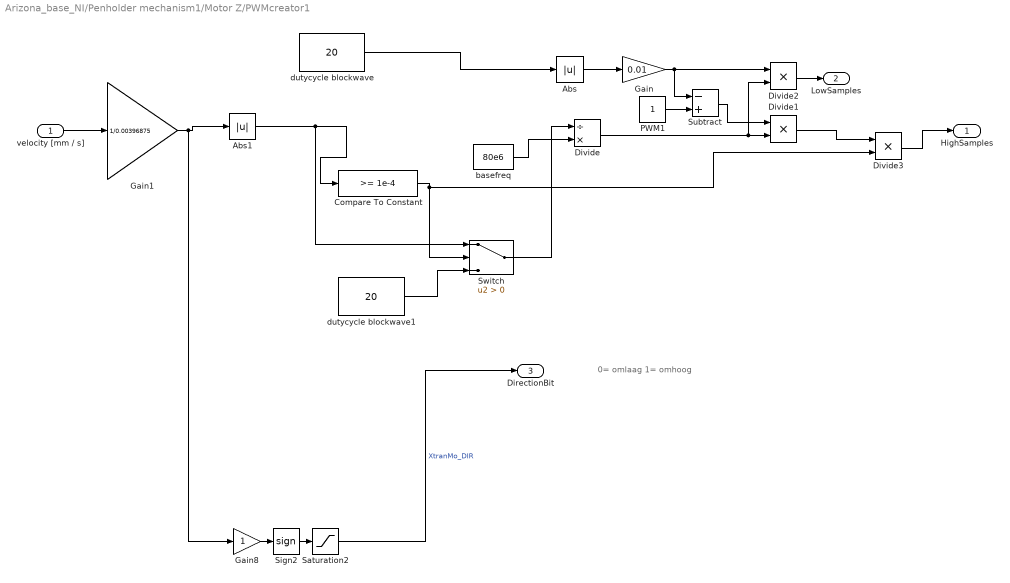
== system Arizona_base_NI/Penholder mechanism1/Motor Z/PWMcreator1 ==
  note: 0= omlaag
      | 1= omhoog
  velocity [mm / s] : Inport
  Abs : Abs
  Abs1 : Abs
  Compare To Constant : simulink/Logic and Bit Operations/Compare To Constant  relop=>=  const=1e-4  OutDataTypeStr=boolean
  Divide : Product  Inputs=/*
  Divide1 : Product  Inputs=**
  Divide2 : Product  Inputs=**
  Divide3 : Product  Inputs=**
  Gain : Gain  Gain=0.01
  Gain1 : Gain  Gain=1/0.00396875
  Gain8 : Gain
  PWM1 : Constant
  Saturation2 : Saturate  UpperLimit=1  LowerLimit=0
  Sign2 : Signum
  Subtract : Sum  Inputs=-+
  Switch : Switch  Criteria=u2 > Threshold
  basefreq : Constant  Value=80e6
  dutycycle blockwave : Constant  Value=20
  dutycycle blockwave1 : Constant  Value=20
  HighSamples : Outport
  LowSamples : Outport  Port=2
  DirectionBit : Outport  Port=3
  wires:
  Divide3/1 -> HighSamples/1
  dutycycle blockwave1/1 -> Switch/3
  Switch/1 -> Divide/1
  Compare To Constant/1 -> Switch/2, Divide3/2
  Gain1/1 -> Gain8/1, Abs1/1
  Abs1/1 -> Switch/1, Compare To Constant/1
  basefreq/1 -> Divide/2
  Gain/1 -> Divide2/1, Subtract/1
  Divide/1 -> Divide2/2, Divide1/2
  Subtract/1 -> Divide1/1
  PWM1/1 -> Subtract/2
  dutycycle blockwave/1 -> Abs/1
  Divide2/1 -> LowSamples/1
  velocity [mm / s]/1 -> Gain1/1
  Divide1/1 -> Divide3/1
  Gain8/1 -> Sign2/1
  Sign2/1 -> Saturation2/1
  Abs/1 -> Gain/1
  Saturation2/1 -> DirectionBit/1  "XtranMo_DIR"

== stateflow chart Arizona_base_NI/Trial control ==
  state TRIAL_FINISHED
    en:
    trialTrigger=0;
    change_color=0;
  state PEN_CHANGING
  state idle
    en:
    trialTrigger = 0;
  state initialization
  state PEN_READY
    en:
    change_color=0;
  state trial
    en:
    trialTrigger = 1;
    timeIndex = 0;
    trialIndex++;
    du:
    timeIndex++;
  idle -> PEN_CHANGING [order 1] : [startPenholder==1 && PenColor == 1]
      | {change_color=6}
  TRIAL_FINISHED -> PEN_CHANGING : [after(0.1,sec)]
      | {change_color=PenColor}
  idle -> PEN_CHANGING [order 2] : [startPenholder==1 && PenColor ~= 1]
      | {change_color = PenColor}
  PEN_CHANGING -> PEN_READY : [after(0.1,sec) && penholder_active==0]
  trial -> TRIAL_FINISHED : %Transition if trial is ended.
      | [TrialDone]
  initialization -> idle : %Transition if initialization is completed.
      | [homingDone]
  (default) -> initialization
  PEN_READY -> idle [order 2] : [startPenholder==0]{change_color=5}
  PEN_READY -> trial [order 1] : %Start ILC trial
      | [startTrial]
  data: homingDone input double; startTrial input double; startPenholder input; trialTrigger output double =0; timeIndex local double =0; N_ref parameter double; trialIndex output double =0; TrialDone input; change_color output double; penholder_active input; PenColor input

== stateflow chart Arizona_base_NI/Homing/Enabled subsystem/Reset/Supervisor ==
  state MOVE_PEN_UP
    entry:
    change_color=5;
  state PEN_READY
    entry:
    change_color=0;
  state MoveToLimitSwitches
    state reset_gantryLeft [parallel]
      settings: executionOrder=1
      state increase_jogspeed
        during:
        jogspeed_xL_reset = max(-0.10,jogspeed_xL_reset - 0.10*Ts/1);
      state stop
        entry:
        jogspeed_xL_reset = 0;
      (default) -> MoveToLimitSwitches.reset_gantryLeft.increase_jogspeed
      MoveToLimitSwitches.reset_gantryLeft.increase_jogspeed -> MoveToLimitSwitches.reset_gantryLeft.stop : [limitswitch_xL]
    state reset_gantryright [parallel]
      settings: executionOrder=2
      state increase_jogspeed
        during:
        jogspeed_xR_reset = max(-0.10,jogspeed_xR_reset - 0.10*Ts/1);
      state stop
        entry:
        jogspeed_xR_reset = 0;
      (default) -> MoveToLimitSwitches.reset_gantryright.increase_jogspeed
      MoveToLimitSwitches.reset_gantryright.increase_jogspeed -> MoveToLimitSwitches.reset_gantryright.stop : [limitswitch_xR]
    state reset_carriage [parallel]
      settings: executionOrder=3
      state increase_jogspeed
        during:
        jogspeed_y_reset = max(-0.25,jogspeed_y_reset - 0.25*Ts/1);
      state stop
        entry:
        jogspeed_y_reset = 0;
      (default) -> MoveToLimitSwitches.reset_carriage.increase_jogspeed
      MoveToLimitSwitches.reset_carriage.increase_jogspeed -> MoveToLimitSwitches.reset_carriage.stop : [limitswitch_y]
  state enablePointToRefs
    entry:
    resetDone = true;
  (default) -> MOVE_PEN_UP
  MOVE_PEN_UP -> PEN_READY : [after(1,sec) && penholder_active==0]
  PEN_READY -> MoveToLimitSwitches
  MoveToLimitSwitches -> enablePointToRefs : [(jogspeed_xL_reset==0) && (jogspeed_xR_reset==0) && (jogspeed_y_reset==0)]
  data: jogspeed_y_reset output double =-0.25*Ts/1; jogspeed_xL_reset output double =-0.10*Ts/1; limitswitch_y input double; limitswitch_xL input double; limitswitch_xR input double; jogspeed_xR_reset output double =-0.10*Ts/1; resetDone output double =0; Ts local double =Ts; penholder_active input; change_color output double

== stateflow chart Arizona_base_NI/Safety/Supervisor ==
  state evaluateSatefy
    state gantryAirbag [parallel]
      settings: executionOrder=3
      state defaultState
        exit:
        enableAirbags = true;
      state backAirbag
        entry:
        current_gantryAirbag = -5;
      state frontAirbag
        entry:
        current_gantryAirbag = 5;
      state stop_gantryAirbag
        entry:
        current_gantryAirbag = 0;
      (default) -> evaluateSatefy.gantryAirbag.defaultState
      evaluateSatefy.gantryAirbag.defaultState -> frontAirbag [order 1] : [homingDone && xNom<0.1075-xInit_end]
      evaluateSatefy.gantryAirbag.defaultState -> backAirbag [order 2] : [homingDone && xNom>1.035-xInit_end-0.1075]
      backAirbag -> stop_gantryAirbag : [velocity_x<=0]
      frontAirbag -> stop_gantryAirbag : [velocity_x>=0]
    state errorAirbag [parallel]
      settings: executionOrder=1
      state defaultState
      state errorStop
        entry:
        enableAirbags = true;
      (default) -> evaluateSatefy.errorAirbag.defaultState
      evaluateSatefy.errorAirbag.defaultState -> errorStop : [abs(error_x)>0.05 || abs(error_y)>0.05 || abs(error_phi)>0.05 || abs(phi)>atan(.01/2.6)]
    state carriageAirbag [parallel]
      settings: executionOrder=2
      state defaultState
        exit:
        enableAirbags = true;
      state leftAirbag
        entry:
        current_carriageAirbag = 5;
      state rightAirbag
        entry:
        current_carriageAirbag = -5;
      state stop_carriageAirbag
        entry:
        current_carriageAirbag = 0;
      (default) -> evaluateSatefy.carriageAirbag.defaultState
      evaluateSatefy.carriageAirbag.defaultState -> leftAirbag [order 1] : [homingDone && yNom<0.19-yInit_end]
      evaluateSatefy.carriageAirbag.defaultState -> rightAirbag [order 2] : [homingDone && yNom>3.2-yInit_end-0.19]
      leftAirbag -> stop_carriageAirbag : [velocity_y>=0]
      rightAirbag -> stop_carriageAirbag : [velocity_y<=0]
  state stopCarriage
    entry:
    stopSimulation = true;
  (default) -> evaluateSatefy
  evaluateSatefy -> stopCarriage : % Stop simulation if the airbags are active with zero current and the velocity is small.
      | [ enableAirbags && current_carriageAirbag == 0 && current_gantryAirbag == 0 && sqrt(velocity_x^2+velocity_y^2)<0.01 ]
  data: xInit_end constant double =xInit(end); yInit_end constant double =yInit(end); homingDone input double; error_y input double =false; yNom input double =false; velocity_y input double =false; error_x input double =false; current_carriageAirbag output double =0; enableAirbags output double =false; xNom input double =false; velocity_x input double =false; error_phi input double =false; current_gantryAirbag output double =0; stopSimulation output double =false; phi input double

== stateflow chart Arizona_base_NI/Penholder mechanism1/Change color Chart ==
  state MOVE_PENHOLDER
    state MAIN [parallel]
      settings: executionOrder=1
      state INITIAL
        entry:
        active=0;
        job=0;
      state IDLE
      state HOMING
      state FINISHED
        entry:
        active=0;
      state GOING_UP
        entry:
        active=1;
      state GOING_DOWN
        entry:
        active=1;
      state ROTATING
      (default) -> MOVE_PENHOLDER.MAIN.INITIAL
      MOVE_PENHOLDER.MAIN.IDLE -> MOVE_PENHOLDER.MAIN.IDLE [order 3] : [job~=change_color ...
          | && change_color==0]
          | {job=change_color}
      MOVE_PENHOLDER.MAIN.INITIAL -> MOVE_PENHOLDER.MAIN.IDLE
      MOVE_PENHOLDER.MAIN.IDLE -> GOING_UP [order 1] : [job ~= change_color && change_color~=0 ...
          | && homingDone ~=0 && change_color~=6]
          | {send(go_up,VERTICAL);job=change_color}
      MOVE_PENHOLDER.MAIN.IDLE -> HOMING [order 4] : [homingDone==0 ...
          | && change_color==5]
          | {send(start_homing,HOME)}
      FINISHED -> MOVE_PENHOLDER.MAIN.IDLE
      MOVE_PENHOLDER.MAIN.IDLE -> GOING_DOWN [order 2] : [job ~= change_color ...
          | && change_color==6]
          | {send(go_down,VERTICAL);job=change_color}
      HOMING -> FINISHED : [homing_done]
      GOING_UP -> FINISHED [order 1] : [is_up && job==5]
      GOING_DOWN -> FINISHED : [is_down]
      GOING_UP -> ROTATING [order 2] : [is_up && job~=5]
          | {send(start_rotate,ROTATION)}
      ROTATING -> GOING_DOWN : [rotate_done && job~=7]
          | {send(go_down,VERTICAL)}
    state VERTICAL [parallel]
      settings: executionOrder=2
      state ALREADY_DOWN
      state DOWN
        entry:
        jogspeed_Z=0;
      state MOVING_UP
        entry:
        jogspeed_Z=1;
      state MOVING_DOWN
        entry:
        jogspeed_Z=-1;
      state INITIAL
      state UP
        entry:
        jogspeed_Z=0;
      state ALREADY_UP
      ALREADY_DOWN -> DOWN : [after(0.1,sec)]{send(is_down,MAIN)}
      DOWN -> ALREADY_DOWN [order 2] : go_down
      DOWN -> MOVE_PENHOLDER.VERTICAL.MOVING_UP [order 1] : go_up
      MOVING_DOWN -> DOWN : [limitSwitch_z_down==1]
          | {send(is_down,MAIN)}
      (default) -> MOVE_PENHOLDER.VERTICAL.INITIAL
      MOVE_PENHOLDER.VERTICAL.INITIAL -> MOVE_PENHOLDER.VERTICAL.MOVING_UP [order 1] : go_up
      MOVE_PENHOLDER.VERTICAL.INITIAL -> MOVING_DOWN [order 2] : go_down
      MOVE_PENHOLDER.VERTICAL.UP -> MOVING_DOWN [order 1] : go_down
      MOVE_PENHOLDER.VERTICAL.MOVING_UP -> MOVE_PENHOLDER.VERTICAL.UP : [limitSwitch_z_up==1]
          | {send(is_up,MAIN)}
      ALREADY_UP -> MOVE_PENHOLDER.VERTICAL.UP : [after(0.1,sec)]{send(is_up,MAIN)}
      MOVE_PENHOLDER.VERTICAL.UP -> ALREADY_UP [order 2] : go_up
    state ROTATION [parallel]
      settings: executionOrder=3
      state INITIAL
        en: color_pos=1;
      state INITIALIZE
        entry:
        rot_change = change_color-color_pos;
      state IDLE
        entry:
        jogspeed_Theta=0;
      state CHECK_ROTATE
      state ARRIVAL
        entry:
        counter=counter-1*sign(counter);
        color_pos = change_color;
      state DEPARTURE
        entry:
        jogspeed_Theta = 1*sign(counter);
      (default) -> MOVE_PENHOLDER.ROTATION.INITIAL
      MOVE_PENHOLDER.ROTATION.INITIAL -> MOVE_PENHOLDER.ROTATION.IDLE : [after(0.1,sec)]
      MOVE_PENHOLDER.ROTATION.IDLE -> INITIALIZE : [start_rotate]
      INITIALIZE -> CHECK_ROTATE [order 1] : [-2<=rot_change && rot_change<=2]
          | {counter = rot_change}
      INITIALIZE -> CHECK_ROTATE [order 3] : [rot_change== 3]{counter =-1}
      INITIALIZE -> CHECK_ROTATE [order 2] : [rot_change==-3]{counter = 1}
      ARRIVAL -> MOVE_PENHOLDER.ROTATION.IDLE [order 1] : [counter==0 && change_color==7]
          | {send(rotate_done,MAIN); color_pos=1}
      ARRIVAL -> MOVE_PENHOLDER.ROTATION.IDLE [order 2] : [counter==0 && change_color~=7]
          | {send(rotate_done,MAIN)}
      CHECK_ROTATE -> DEPARTURE : [counter~=0]
      DEPARTURE -> ARRIVAL : [after(1,sec) && ...
          | limitSwitch_Theta==1]
      ARRIVAL -> DEPARTURE [order 3] : [counter~=0]
    state HOME [parallel]
      settings: executionOrder=4
      state MOVING_UP
        entry:
        jogspeed_Z=1;
      state INITIAL
      state UP
        entry:
        jogspeed_Z=0;
      state DONE
        entry:
        jogspeed_Theta=0;
      state ROTATE
        entry:
        jogspeed_Theta=1;
      (default) -> MOVE_PENHOLDER.HOME.INITIAL
      MOVE_PENHOLDER.HOME.INITIAL -> MOVE_PENHOLDER.HOME.MOVING_UP : [start_homing]
      DONE -> MOVE_PENHOLDER.HOME.INITIAL : {send(homing_done,MAIN)}
      MOVE_PENHOLDER.HOME.MOVING_UP -> MOVE_PENHOLDER.HOME.UP : [limitSwitch_z_up==1]
      MOVE_PENHOLDER.HOME.UP -> DONE [order 1] : [limitSwitch_Theta==1]
      MOVE_PENHOLDER.HOME.UP -> ROTATE [order 2] : [after(0.1,sec) ...
          | && limitSwitch_Theta~=1]
      ROTATE -> DONE : [after(0.1,sec) ...
          | && limitSwitch_Theta==1]
  (default) -> MOVE_PENHOLDER
  data: change_color input; limitSwitch_z_up input; limitSwitch_z_down input; limitSwitch_Theta input; jogspeed_Z output; jogspeed_Theta output; counter local; active output; job local; rot_change local; color_pos local; homingDone input
  events: is_down local FUNCTION_CALL_EVENT; is_up local FUNCTION_CALL_EVENT; go_up local FUNCTION_CALL_EVENT; go_down local FUNCTION_CALL_EVENT; start_rotate local FUNCTION_CALL_EVENT; rotate_done local FUNCTION_CALL_EVENT; start_homing local FUNCTION_CALL_EVENT; homing_done local FUNCTION_CALL_EVENT
